simulink model "commbluetoothfduplex"  (R2018b)
settings: Solver=VariableStepDiscrete  StartTime=0.0  StopTime=2.7  RelTol=1e-3  EnableMultiTasking=on
PostLoadFcn:
  | % set variant-control variable; not as a field of the params structure
  | assignin('base', 'bluetoothChannelID', 3); % 3 --> init to 'AWGN and 802.11b'
InitFcn:
  | commbluetoothfduplex_init;
libraries: commrflib2 x15, commchan3 x4, commbluetoothfduplex_lib x3, commblksprivate x1, dspsrcs4 x1
Description:
  | Bluetooth(R) Full Duplex Voice and Data Transmission
settings Model: Creator=The MathWorks, Inc.  LastModifiedBy=Aviya
settings Model: ModifiedComment=|
  | stuartm -- Fri Jul 20 12:58:27 2001 -- Version 1.201
  | Fix for R12.1. Changed CPM modulator. Replaced enable subsystems in channel with "switch case".
settings Model: ModifiedHistory=|
  | stuartm -- Fri Jul 20 12:58:27 2001 -- Version 1.201
  | Fix for R12.1. Changed CPM modulator. Replaced enable subsystems in channel with "switch case".
  | 
  | 
  | stuartm -- Sun Jul 08 13:59:13 2001 -- Version 1.172
  | Added gain mask at output of transmitter to run it off after 374 bits.
  | 
  | stuartm -- Sun Jul 08 13:53:19 2001 -- Version 1.171
  | Changed hop generator to randint block. Put zero padiing back to before transmitter.
  | 
  | 
  | Started with bluetooth_voice2. Move zero pad from input to output of transmitter. Now only transmits 374 bits
  | 
  | Added channel option
settings DataIOCC: LimitDataPoints=on  SaveFormat=Array  SaveOutput=off  SaveTime=off  SignalLoggingName=sigsOut
settings OptimizationCC: BlockReduction=off  BooleanDataType=off  OptimizeBlockIOStorage=off  BufferReuse=off  GlobalBufferReuse=off  ExpressionFolding=off  ExpressionDepthLimit=2147483647  LocalBlockOutputs=off  InitFltsAndDblsToZero=on  EfficientMapNaN2IntZero=off  LifeSpan=inf  OptimizeDataStoreBuffers=off  BusAssignmentInplaceUpdate=off
settings DebuggingCC: SaveWithParameterizedLinksMsg=none  UnderspecifiedInitializationDetection=Classic  MergeDetectMultiDrivingBlocksExec=none  SignalResolutionControl=TryResolveAllWithWarning  MultiTaskDSMMsg=warning  MultiTaskCondExecSysMsg=none  FcnCallInpInsideContextMsg=warning  AllowSymbolicDim=off  StateNameClashWarn=warning  SFUnexpectedBacktrackingDiag=warning  SFNoUnconditionalDefaultTransitionDiag=warning  SFUnreachableExecutionPathDiag=none  SFExecutionAtInitializationDiag=none
settings HardwareCC: ProdBitPerPointer=32  ProdBitPerSizeT=32  ProdBitPerPtrDiffT=32  ProdLargestAtomicFloat=None  ProdIntDivRoundTo=Undefined  ProdEndianess=Unspecified  ProdWordSize=32  ProdHWDeviceType=32-bit Generic  TargetUnknown=on
settings ModelReferenceCC: PropagateSignalLabelsOutOfModel=off
settings SFSimCC: SimUseLocalCustomCode=off  SimParseCustomCode=off
settings RTWCC: Description=Generic Real-Time Target  RTWUseLocalCustomCode=off
settings CodeAppCC: StateflowObjectComments=on
settings GRTTargetCC: TargetFcnLib=ansi_tfl_tmw.mat  TargetLangStandard=C89/C90 (ANSI)  GeneratePreprocessorConditionals=Disable all  CombineOutputUpdateFcns=off  GRTInterface=on
settings ConfigComp: CovMetricSettings=dw  CovHtmlReporting=on  CovSaveCumulativeToWorkspaceVar=on  CovSaveSingleToWorkspaceVar=on  CovExternalEMLEnable=off  CovSFcnEnable=off

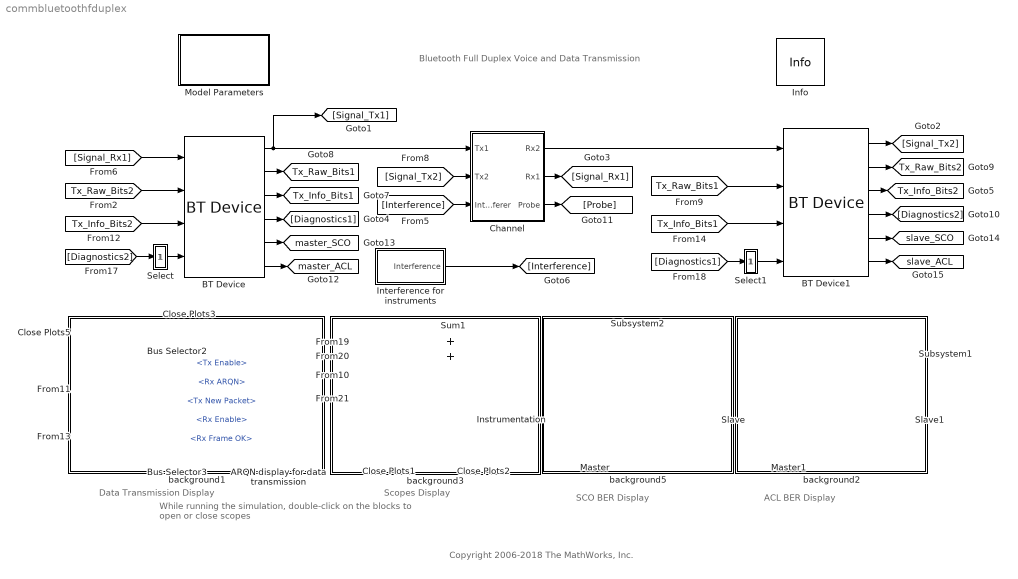
== system commbluetoothfduplex ==
  note: Bluetooth Full Duplex
      |  Voice and Data Transmission
  note: Scopes Display
  note: Data Transmission Display
  note: SCO BER Display
  note: ACL BER Display
  note: While running the simulation, double-click on the blocks to
      | open or close scopes
  note: Copyright 2006-2018 The MathWorks, Inc.
  ARQN display for data transmission : Scope  NumInputPorts=5
  BT Device : commbluetoothfduplex_lib/BT Device  ID=1  Device_Type=Master  mask_packet_type=HV1  Slot_Pair=1&2  Input_File_Name=commbluetoothfduplex_input1.wav
      settings: AttributesFormatString=Device %<ID>: %<Device_Type>  SourceProductName=Communications Toolbox  SourceProductBaseCode=CM
  BT Device1 : commbluetoothfduplex_lib/BT Device  ID=2  Device_Type=Slave  mask_packet_type=HV1  Slot_Pair=1&2  Input_File_Name=commbluetoothfduplex_input2.wav
      settings: AttributesFormatString=Device %<ID>: %<Device_Type>  SourceProductName=Communications Toolbox  SourceProductBaseCode=CM
  Bus Selector2 : BusSelector  OutputSignals=Tx Enable,Rx ARQN,Tx New Packet
  Bus Selector3 : BusSelector  OutputSignals=Rx Enable,Rx Frame OK
  Channel : Subsystem  Variant=on
      settings: AttributesFormatString=%<BlockChoice>
  Close Plots1 : Subsystem
      settings: OpenFcn=|
      | open_system('commbluetoothfduplex/Instrumentation/Subsystem/Spectrum Analyzer');
      | open_system('commbluetoothfduplex/Instrumentation/Subsystem/Timing Diagram');
      mask Display: disp('Open Scopes');
  Close Plots2 : Subsystem
      settings: OpenFcn=|
      | close_system('commbluetoothfduplex/Instrumentation/Subsystem/Spectrum Analyzer');
      | close_system('commbluetoothfduplex/Instrumentation/Subsystem/Timing Diagram');
      mask Display: disp('Close Scopes');
  Close Plots3 : Subsystem
      settings: OpenFcn=set_param([gcs '/ARQN display for data transmission'],'Open','off');
      mask Display: disp('Close Scopes');
  Close Plots5 : Subsystem
      settings: OpenFcn=set_param([gcs '/ARQN display for data transmission'],'Open','on');
      mask Display: disp('Open Scopes');
  Info : commblksprivate/Info  SystemSampleTime=-1
      settings: SourceProductName=Communications Toolbox  SourceProductBaseCode=CM
  Instrumentation : Subsystem  TreatAsAtomicUnit=on  mask(Instrumentation){}
  Interference for instruments : Subsystem  Variant=on
      settings: AttributesFormatString=%<BlockChoice>
  Master : Display
      settings: Decimation=3
  Master1 : Display
      settings: Decimation=3
  Model Parameters : Subsystem  mask(Model Parameters){channel_type=AWGN and 802.11b, packet_type=HV1, slot_pair=1&2}
      mask prompts: channel_type "Channel type"; slot_pair "Initial Slot Pair for HV2 or HV3"
      mask help: Configures both devices to specified system parameters. Takes extra initialization time. EsNo is defined in the MATLAB workspace. Default is 18dB.
      mask init:
      | commbluetoothfduplex_init_block;
      settings: AttributesFormatString=Channel type: %<channel_type>\nPacket Type: %<packet_type>\nInitial Slot Pair: %<slot_pair>
      mask Help: helpview(commdhelp);
      mask TypeOptions channel_type: None | AWGN | AWGN and 802.11b
      mask TypeOptions packet_type: DM1 | HV1 | HV2 | HV3 | SCORT
      mask TypeOptions slot_pair: 1&2 | 3&4 | 5&6
      mask Display: disp('Model\nParameters');
  Select : Subsystem
      mask Display: disp('')
  Select1 : Subsystem
      mask Display: disp('')
  Slave : Display
      settings: Decimation=3
  Slave1 : Display
      settings: Decimation=3
  Subsystem1 : Subsystem
      mask Display: disp('ACL_BER Display\n Master                 Slave');
  Subsystem2 : Subsystem
      mask Display: disp('SCO_BER Display\n Master                  Slave');
  Sum1 : Sum  SaturateOnIntegerOverflow=on  InputSameDT=on  OutDataTypeStr=Inherit: Same as first input
  background1 : Subsystem
      mask Display: disp('')
  background2 : Subsystem
      mask Display: disp('')
  background3 : Subsystem
      mask Display: disp('')
  background5 : Subsystem
      mask Display: disp('')
  tag scope: Tx_Info_Bits1=global, Tx_Info_Bits2=global, Tx_Raw_Bits1=global, Tx_Raw_Bits2=global, master_ACL=global, master_SCO=global, slave_ACL=global, slave_SCO=global
  wires:
  Interference for instruments/1(Interference) -> [Interference]
  Select/1(Out1) -> BT Device/4
  BT Device1/1 -> [Signal_Tx2]
  Select1/1(Out1) -> BT Device1/4
  BT Device/2 -> [Tx_Raw_Bits1]
  BT Device/3 -> [Tx_Info_Bits1]
  [Tx_Raw_Bits1] -> BT Device1/2
  [Tx_Info_Bits1] -> BT Device1/3
  [Tx_Raw_Bits2] -> BT Device/2
  [Tx_Info_Bits2] -> BT Device/3
  BT Device1/2 -> [Tx_Raw_Bits2]
  BT Device1/3 -> [Tx_Info_Bits2]
  [Diagnostics2] -> Select/1(In1)
  [Diagnostics1] -> Select1/1(In1)
  [Interference] -> Channel/3(Interferer)
  [Signal_Rx1] -> BT Device/1
  [Signal_Tx2] -> Channel/2(Tx2)
  Channel/1(Rx2) -> BT Device1/1
  Channel/2(Rx1) -> [Signal_Rx1]
  Channel/3(Probe) -> [Probe]
  BT Device/1 -> Channel/1(Tx1), [Signal_Tx1]
  BT Device/5 -> [master_SCO]
  BT Device1/5 -> [slave_SCO]
  Subsystem2/1(Out1) -> Master/1
  Subsystem2/2(Out2) -> Slave/1
  Bus Selector2/1 -> ARQN display for data transmission/1  "<Tx Enable>"
  Bus Selector2/2 -> ARQN display for data transmission/2  "<Rx ARQN>"
  Bus Selector2/3 -> ARQN display for data transmission/3  "<Tx New Packet>"
  Bus Selector3/1 -> ARQN display for data transmission/4  "<Rx Enable>"
  Bus Selector3/2 -> ARQN display for data transmission/5  "<Rx Frame OK>"
  [Diagnostics1] -> Bus Selector2/1
  [Diagnostics2] -> Bus Selector3/1
  [Probe] -> Instrumentation/3(Rx)
  [Signal_Tx1] -> Sum1/1
  [Signal_Tx2] -> Sum1/2
  Sum1/1 -> Instrumentation/1(Tx)
  [Interference] -> Instrumentation/2(Tx_802)
  BT Device/4 -> [Diagnostics1]
  BT Device1/4 -> [Diagnostics2]
  Subsystem1/1(Out1) -> Master1/1
  Subsystem1/2(Out2) -> Slave1/1
  BT Device/6 -> [master_ACL]
  BT Device1/6 -> [slave_ACL]

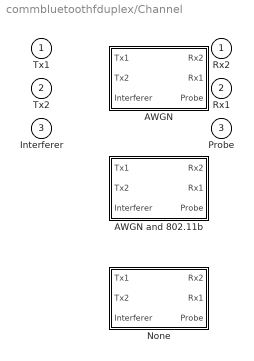
== system commbluetoothfduplex/Channel ==
  Tx1 : Inport
  Tx2 : Inport  Port=2
  Interferer : Inport  Port=3
  AWGN : Subsystem  VariantControl=bluetoothChannelID == 2
  AWGN and 802.11b : Subsystem  VariantControl=bluetoothChannelID == 3
  None : Subsystem  VariantControl=bluetoothChannelID == 1
  Rx2 : Outport
  Rx1 : Outport  Port=2
  Probe : Outport  Port=3

== system commbluetoothfduplex/Close Plots1 ==

== system commbluetoothfduplex/Close Plots2 ==

== system commbluetoothfduplex/Close Plots3 ==

== system commbluetoothfduplex/Close Plots5 ==

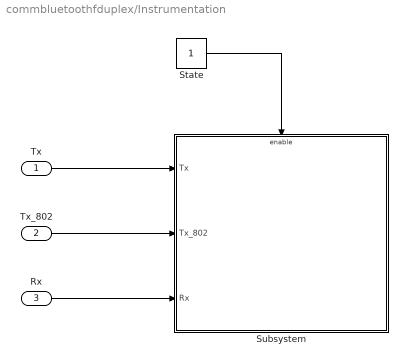
== system commbluetoothfduplex/Instrumentation ==
  Tx : Inport
  Tx_802 : Inport  Port=2
  Rx : Inport  Port=3
  State : Constant
  Subsystem : Subsystem  TreatAsAtomicUnit=on
  wires:
  State/1 -> Subsystem/Enable
  Tx_802/1 -> Subsystem/2(Tx_802)
  Tx/1 -> Subsystem/1(Tx)
  Rx/1 -> Subsystem/3(Rx)

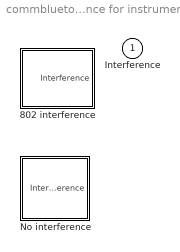
== system commbluetoothfduplex/Interference for instruments ==
  802 interference : Subsystem  VariantControl=bluetoothChannelID == 3
  No interference : Subsystem  VariantControl=bluetoothChannelID < 3
  Interference : Outport

== system commbluetoothfduplex/Model Parameters ==

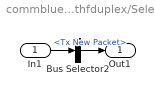
== system commbluetoothfduplex/Select ==
  In1 : Inport
  Bus Selector2 : BusSelector  OutputSignals=Tx New Packet
  Out1 : Outport
  wires:
  In1/1 -> Bus Selector2/1
  Bus Selector2/1 -> Out1/1  "<Tx New Packet>"

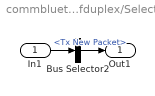
== system commbluetoothfduplex/Select1 ==
  In1 : Inport
  Bus Selector2 : BusSelector  OutputSignals=Tx New Packet
  Out1 : Outport
  wires:
  Bus Selector2/1 -> Out1/1  "<Tx New Packet>"
  In1/1 -> Bus Selector2/1

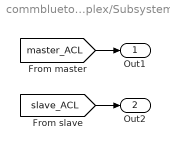
== system commbluetoothfduplex/Subsystem1 ==
  Out1 : Outport
  Out2 : Outport  Port=2
  wires:
  [master_ACL] -> Out1/1
  [slave_ACL] -> Out2/1

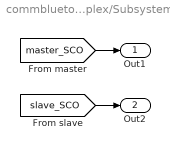
== system commbluetoothfduplex/Subsystem2 ==
  Out1 : Outport
  Out2 : Outport  Port=2
  wires:
  [slave_SCO] -> Out2/1
  [master_SCO] -> Out1/1

== system commbluetoothfduplex/background1 ==

== system commbluetoothfduplex/background2 ==

== system commbluetoothfduplex/background3 ==

== system commbluetoothfduplex/background5 ==

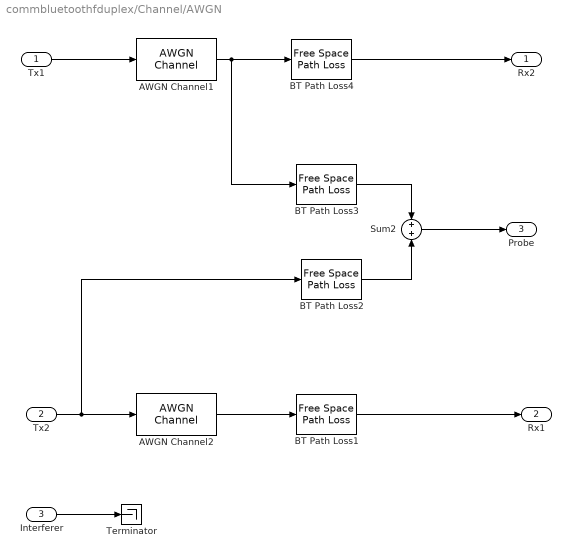
== system commbluetoothfduplex/Channel/AWGN ==
  Tx1 : Inport
  Tx2 : Inport  Port=2
  Interferer : Inport  Port=3
  AWGN Channel1 : commchan3/AWGN Channel  InputProcessing=Columns as channels (frame based)  seed=bluetooth_fd.awgn_channel_seed  noiseMode="Signal to noise ratio  (Es/No)"  EbNodB=10  EsNodB=bluetooth_fd.EsNo  SNRdB=10  bitsPerSym=1  Ps=0.001  Tsym=1e-6  variance=1
      settings: SourceProductName=Communications Toolbox
  AWGN Channel2 : commchan3/AWGN Channel  InputProcessing=Columns as channels (frame based)  seed=bluetooth_fd.awgn_channel_seed  noiseMode="Signal to noise ratio  (Es/No)"  EbNodB=10  EsNodB=bluetooth_fd.EsNo  SNRdB=10  bitsPerSym=1  Ps=0.001  Tsym=1e-6  variance=1
      settings: SourceProductName=Communications Toolbox
  BT Path Loss1 : commrflib2/Free Space Path Loss  mode=Distance and Frequency  dB=10  d=0.001  fc=2400
      settings: AttributesFormatString=Distance: %<d>km  SourceProductName=Communications Toolbox  SourceProductBaseCode=CM
  BT Path Loss2 : commrflib2/Free Space Path Loss  mode=Distance and Frequency  dB=10  d=0.0005  fc=2400
      settings: AttributesFormatString=Distance: %<d>km  SourceProductName=Communications Toolbox  SourceProductBaseCode=CM
  BT Path Loss3 : commrflib2/Free Space Path Loss  mode=Distance and Frequency  dB=10  d=0.0005  fc=2400
      settings: AttributesFormatString=Distance: %<d>km  SourceProductName=Communications Toolbox  SourceProductBaseCode=CM
  BT Path Loss4 : commrflib2/Free Space Path Loss  mode=Distance and Frequency  dB=10  d=0.001  fc=2400
      settings: AttributesFormatString=Distance: %<d>km  SourceProductName=Communications Toolbox  SourceProductBaseCode=CM
  Sum2 : Sum  SaturateOnIntegerOverflow=on
  Terminator : Terminator
  Rx2 : Outport
  Rx1 : Outport  Port=2
  Probe : Outport  Port=3
  wires:
  AWGN Channel1/1 -> BT Path Loss3/1, BT Path Loss4/1
  Tx1/1 -> AWGN Channel1/1
  Interferer/1 -> Terminator/1
  Tx2/1 -> AWGN Channel2/1, BT Path Loss2/1
  AWGN Channel2/1 -> BT Path Loss1/1
  BT Path Loss4/1 -> Rx2/1
  BT Path Loss1/1 -> Rx1/1
  Sum2/1 -> Probe/1
  BT Path Loss3/1 -> Sum2/1
  BT Path Loss2/1 -> Sum2/2

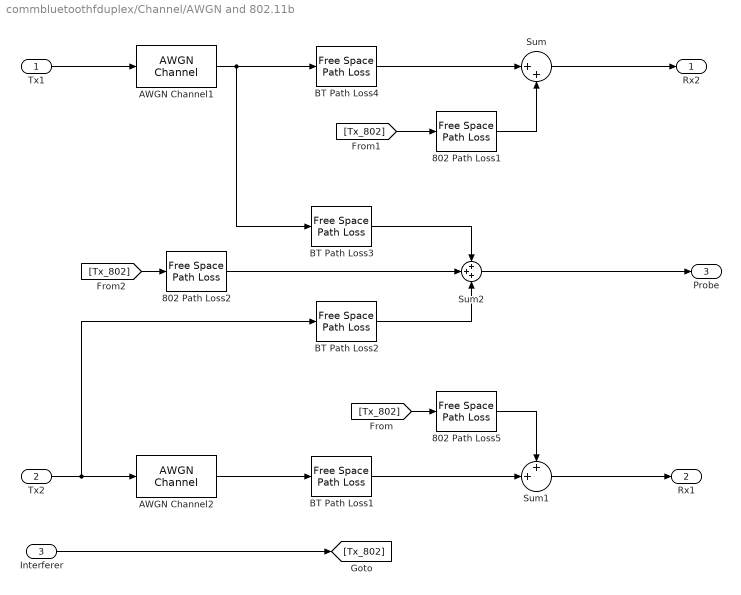
== system commbluetoothfduplex/Channel/AWGN and 802.11b ==
  Tx1 : Inport
  Tx2 : Inport  Port=2
  Interferer : Inport  Port=3
  802 Path Loss1 : commrflib2/Free Space Path Loss  mode=Distance and Frequency  dB=10  d=0.001  fc=2400
      settings: AttributesFormatString=Distance: %<d>km  SourceProductName=Communications Toolbox  SourceProductBaseCode=CM
  802 Path Loss2 : commrflib2/Free Space Path Loss  mode=Distance and Frequency  dB=10  d=0.0005  fc=2400
      settings: AttributesFormatString=Distance: %<d>km  SourceProductName=Communications Toolbox  SourceProductBaseCode=CM
  802 Path Loss5 : commrflib2/Free Space Path Loss  mode=Distance and Frequency  dB=10  d=0.001  fc=2400
      settings: AttributesFormatString=Distance: %<d>km  SourceProductName=Communications Toolbox  SourceProductBaseCode=CM
  AWGN Channel1 : commchan3/AWGN Channel  InputProcessing=Columns as channels (frame based)  seed=bluetooth_fd.awgn_channel_seed  noiseMode="Signal to noise ratio  (Es/No)"  EbNodB=10  EsNodB=bluetooth_fd.EsNo  SNRdB=10  bitsPerSym=1  Ps=0.001  Tsym=1e-6  variance=1
      settings: SourceProductName=Communications Toolbox
  AWGN Channel2 : commchan3/AWGN Channel  InputProcessing=Columns as channels (frame based)  seed=bluetooth_fd.awgn_channel_seed  noiseMode="Signal to noise ratio  (Es/No)"  EbNodB=10  EsNodB=bluetooth_fd.EsNo  SNRdB=10  bitsPerSym=1  Ps=0.001  Tsym=1e-6  variance=1
      settings: SourceProductName=Communications Toolbox
  BT Path Loss1 : commrflib2/Free Space Path Loss  mode=Distance and Frequency  dB=10  d=0.001  fc=2400
      settings: AttributesFormatString=Distance: %<d>km  SourceProductName=Communications Toolbox  SourceProductBaseCode=CM
  BT Path Loss2 : commrflib2/Free Space Path Loss  mode=Distance and Frequency  dB=10  d=0.0005  fc=2400
      settings: AttributesFormatString=Distance: %<d>km  SourceProductName=Communications Toolbox  SourceProductBaseCode=CM
  BT Path Loss3 : commrflib2/Free Space Path Loss  mode=Distance and Frequency  dB=10  d=0.0005  fc=2400
      settings: AttributesFormatString=Distance: %<d>km  SourceProductName=Communications Toolbox  SourceProductBaseCode=CM
  BT Path Loss4 : commrflib2/Free Space Path Loss  mode=Distance and Frequency  dB=10  d=0.001  fc=2400
      settings: AttributesFormatString=Distance: %<d>km  SourceProductName=Communications Toolbox  SourceProductBaseCode=CM
  Sum : Sum  Inputs=|++  SaturateOnIntegerOverflow=on
  Sum1 : Sum  Inputs=++|  SaturateOnIntegerOverflow=on
  Sum2 : Sum  Inputs=+++  SaturateOnIntegerOverflow=on
  Rx2 : Outport
  Rx1 : Outport  Port=2
  Probe : Outport  Port=3
  wires:
  AWGN Channel1/1 -> BT Path Loss3/1, BT Path Loss4/1
  Tx1/1 -> AWGN Channel1/1
  Interferer/1 -> [Tx_802]
  Tx2/1 -> AWGN Channel2/1, BT Path Loss2/1
  AWGN Channel2/1 -> BT Path Loss1/1
  BT Path Loss4/1 -> Sum/1
  Sum1/1 -> Rx1/1
  Sum/1 -> Rx2/1
  BT Path Loss1/1 -> Sum1/2
  [Tx_802] -> 802 Path Loss5/1
  Sum2/1 -> Probe/1
  BT Path Loss3/1 -> Sum2/1
  [Tx_802] -> 802 Path Loss1/1
  BT Path Loss2/1 -> Sum2/3
  [Tx_802] -> 802 Path Loss2/1
  802 Path Loss5/1 -> Sum1/1
  802 Path Loss1/1 -> Sum/2
  802 Path Loss2/1 -> Sum2/2

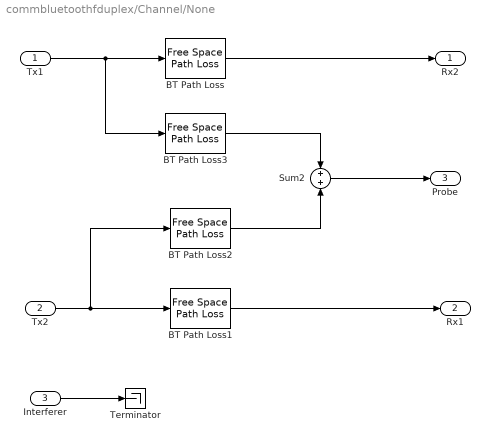
== system commbluetoothfduplex/Channel/None ==
  Tx1 : Inport
  Tx2 : Inport  Port=2
  Interferer : Inport  Port=3
  BT Path Loss : commrflib2/Free Space Path Loss  mode=Distance and Frequency  dB=10  d=0.001  fc=2400
      settings: AttributesFormatString=Distance: %<d>km  SourceProductName=Communications Toolbox  SourceProductBaseCode=CM
  BT Path Loss1 : commrflib2/Free Space Path Loss  mode=Distance and Frequency  dB=10  d=0.001  fc=2400
      settings: AttributesFormatString=Distance: %<d>km  SourceProductName=Communications Toolbox  SourceProductBaseCode=CM
  BT Path Loss2 : commrflib2/Free Space Path Loss  mode=Distance and Frequency  dB=10  d=0.0005  fc=2400
      settings: AttributesFormatString=Distance: %<d>km  SourceProductName=Communications Toolbox  SourceProductBaseCode=CM
  BT Path Loss3 : commrflib2/Free Space Path Loss  mode=Distance and Frequency  dB=10  d=0.0005  fc=2400
      settings: AttributesFormatString=Distance: %<d>km  SourceProductName=Communications Toolbox  SourceProductBaseCode=CM
  Sum2 : Sum  SaturateOnIntegerOverflow=on
  Terminator : Terminator
  Rx2 : Outport
  Rx1 : Outport  Port=2
  Probe : Outport  Port=3
  wires:
  Tx1/1 -> BT Path Loss/1, BT Path Loss3/1
  Interferer/1 -> Terminator/1
  BT Path Loss/1 -> Rx2/1
  Tx2/1 -> BT Path Loss1/1, BT Path Loss2/1
  BT Path Loss1/1 -> Rx1/1
  Sum2/1 -> Probe/1
  BT Path Loss3/1 -> Sum2/1
  BT Path Loss2/1 -> Sum2/2

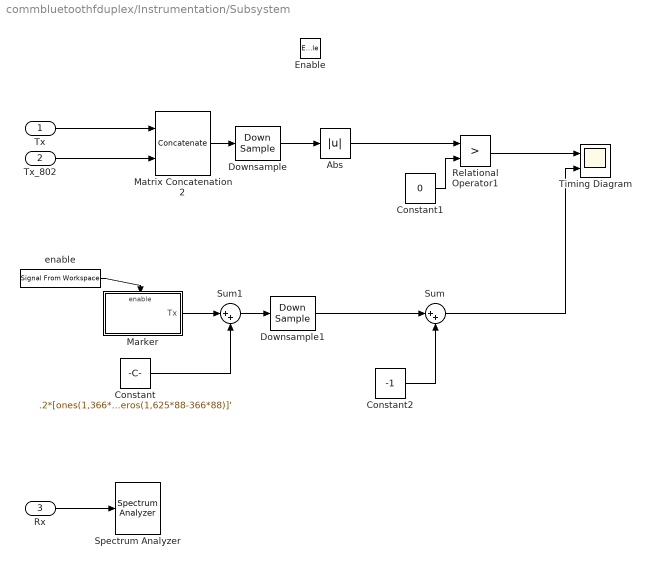
== system commbluetoothfduplex/Instrumentation/Subsystem ==
  Tx : Inport
  Tx_802 : Inport  Port=2
  Rx : Inport  Port=3
  Enable : EnablePort  PropagateVarSize=During execution
  Abs : Abs  SaturateOnIntegerOverflow=on
  Constant : Constant  Value=.2*[ones(1,366*88) zeros(1,625*88-366*88)]'  VectorParams1D=off  SampleTime=625e-6
  Constant1 : Constant  Value=0
  Constant2 : Constant  Value=-1
  Downsample : DownSample  N=125
  Downsample1 : DownSample  N=125
  Marker : Subsystem  TreatAsAtomicUnit=on
  Matrix Concatenation2 : Concatenate  Mode=Multidimensional array  ConcatenateDimension=2
  Relational Operator1 : RelationalOperator  Operator=>  RndMeth=Nearest  InputSameDT=on
  Spectrum Analyzer : SpectrumAnalyzer
  Sum : Sum  Inputs=|++  SaturateOnIntegerOverflow=on  InputSameDT=on  OutDataTypeStr=Inherit: Same as first input
  Sum1 : Sum  Inputs=|++  SaturateOnIntegerOverflow=on  InputSameDT=on  OutDataTypeStr=Inherit: Same as first input
  Timing Diagram : Scope  NumInputPorts=2
  enable : dspsrcs4/Signal From Workspace  X=[1 0 0 0 0 0]  Ts=625e-6  nsamps=1  OutputAfterFinalValue=Cyclic repetition  ignoreOrWarnInputAndFrameLengths=off  OutputFrames=on
  wires:
  Constant/1 -> Sum1/2
  Sum1/1 -> Downsample1/1
  Marker/1(Tx) -> Sum1/1
  Downsample1/1 -> Sum/1
  Constant2/1 -> Sum/2
  Relational Operator1/1 -> Timing Diagram/1
  Sum/1 -> Timing Diagram/2
  enable/1 -> Marker/Enable
  Matrix Concatenation2/1 -> Downsample/1
  Tx/1 -> Matrix Concatenation2/1
  Tx_802/1 -> Matrix Concatenation2/2
  Abs/1 -> Relational Operator1/1
  Constant1/1 -> Relational Operator1/2
  Rx/1 -> Spectrum Analyzer/1
  Downsample/1 -> Abs/1

== system commbluetoothfduplex/Interference for instruments/802 interference ==
  802.11b Transmitter : commbluetoothfduplex_lib/802.11b Transmitter  On=on  rate=50  m=(192+1024*8)*1e-6 %(preamble size + 1024 bytes) x bit rate  v=0  power=16  Freq_Number=39  rate_seed=bluetooth_fd.rate_802_seed  awgn_seed=bluetooth_fd.awgn_802_seed
      settings: SourceProductName=Communications Toolbox  SourceProductBaseCode=CM
  Interference : Outport
  wires:
  802.11b Transmitter/1 -> Interference/1

== system commbluetoothfduplex/Interference for instruments/No interference ==
  Constant : Constant  Value=zeros(55000,1)  VectorParams1D=off  SampleTime=1/1600
  Interference : Outport
  wires:
  Constant/1 -> Interference/1

== system commbluetoothfduplex/Instrumentation/Subsystem/Marker ==
  Enable : EnablePort  PropagateVarSize=During execution
  Constant : Constant  Value=.1*[ones(1,366*88) zeros(1,625*88-366*88)]'  VectorParams1D=off  SampleTime=625e-6
  Tx : Outport  OutputWhenDisabled=reset  InitialOutput=0
  wires:
  Constant/1 -> Tx/1
